simulink model "ex6discreto"  (R2015a)
settings: Solver=ode45  StartTime=0.0  StopTime=10  RelTol=1e-3
values from neighbouring files (symbols this model uses):
  G = 1/(s*(s+c))    [ex6.m]
  Ts = 1/fs    (= 0.05)    [ex6.m]    (also in matlab.mat; sim_ex6.m = C.Ts)
settings Model: Creator=BPeixoto  LastModifiedBy=BPeixoto

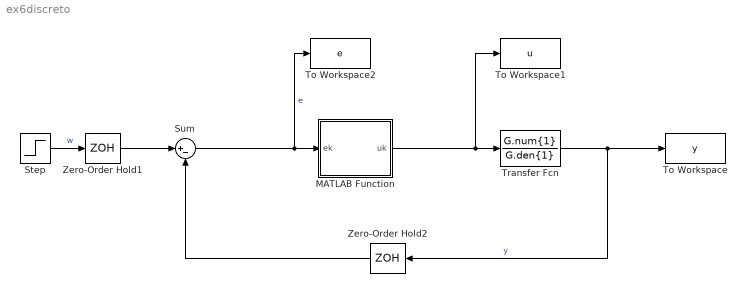
== system ex6discreto ==
  MATLAB Function : MATLAB Function  TreatAsAtomicUnit=on
  Step : Step  Time=0  SampleTime=Ts
  Sum : Sum  Inputs=|+-
  To Workspace : ToWorkspace  VariableName=y  SaveFormat=Structure With Time  SampleTime=-1
  To Workspace1 : ToWorkspace  VariableName=u  SaveFormat=Structure With Time  SampleTime=-1
  To Workspace2 : ToWorkspace  VariableName=e  SaveFormat=Structure With Time  SampleTime=-1
  Transfer Fcn : TransferFcn  Numerator=G.num{1}  Denominator=G.den{1}
  Zero-Order Hold1 : ZeroOrderHold  SampleTime=Ts
  Zero-Order Hold2 : ZeroOrderHold  SampleTime=Ts
  wires:
  Transfer Fcn/1 -> Zero-Order Hold2/1, To Workspace/1  "y"
  MATLAB Function/1(uk) -> Transfer Fcn/1, To Workspace1/1
  Sum/1 -> To Workspace2/1, MATLAB Function/1(ek)  "e"
  Step/1 -> Zero-Order Hold1/1  "w"
  Zero-Order Hold1/1 -> Sum/1
  Zero-Order Hold2/1 -> Sum/2

== matlab function ex6discreto/MATLAB Function ==
  data: ek input; uk output; params parameter
% @author: Bruno Peixoto
% Efetua o controle de posicao de um motor DC
% por transformacao de tustin
function uk = controlador(ek, params)
    persistent e_ant;
    persistent u_ant;
    
     % Primeira execucao
     if(isempty(e_ant))
         e_ant = [0, 0];
     end
     
     if(isempty(u_ant))
         u_ant = 0;
     end
    
    % Parâmetros do controlador
    b0 = params.b0;
    b1 = params.b1;
    a0 = params.a0;
    a1 = params.a1;

    % Atualizacao do erro
    e_ant(1) = e_ant(2);
    e_ant(2) = ek;
    
    % Valores para controle
    ek_1 = e_ant(1);
    ek = e_ant(2);
    uk_1 = u_ant;

    % Acao de controle
    uk = (b0/a0)*ek + (b1/a0)*ek_1 - (a1/a0)*uk_1;

    % Atualizacao da acao de controle
    u_ant = uk;
end
